simulink library "inverter_model"  (R2024b)
settings: Solver=VariableStepAuto  StartTime=0.0  StopTime=10.0  RelTol=1e-3
settings Model: Creator=jessi  LastModifiedBy=jessi

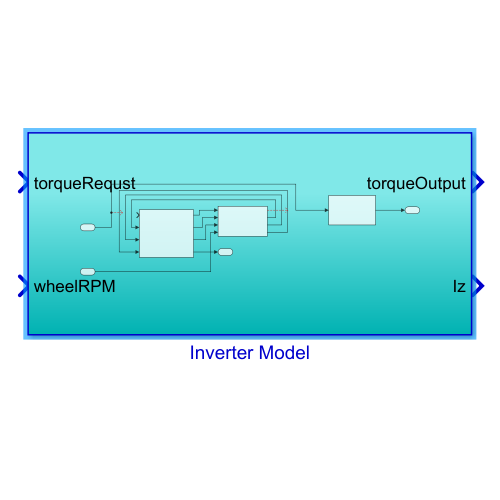
[thumbnail: Simulink's stored preview of the top-level diagram]
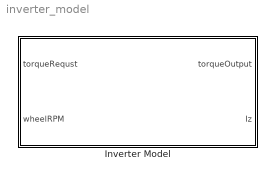
== system inverter_model ==
  Inverter Model : Subsystem

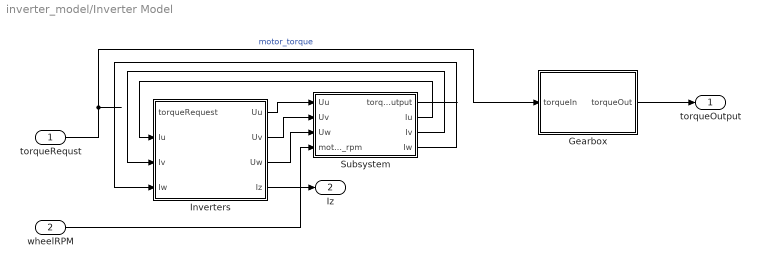
== system inverter_model/Inverter Model ==
  torqueRequst : Inport
  wheelRPM : Inport  Port=2
  Gearbox : Subsystem
  Inverters : Subsystem
  Subsystem : Subsystem
  torqueOutput : Outport
  Iz : Outport  Port=2
  wires:
  torqueRequst/1 -> Gearbox/1(torqueIn)  "motor_torque"
  Subsystem/1(torqueOutput) -> ?
  Inverters/1(Uu) -> Subsystem/1(Uu)
  Inverters/2(Uv) -> Subsystem/2(Uv)
  Inverters/3(Uw) -> Subsystem/3(Uw)
  Subsystem/2(Iu) -> Inverters/2(Iu)
  Subsystem/3(Iv) -> Inverters/3(Iv)
  Subsystem/4(Iw) -> Inverters/4(Iw)
  Inverters/4(Iz) -> Iz/1
  Gearbox/1(torqueOut) -> torqueOutput/1
  wheelRPM/1 -> Subsystem/4(motor_rpm)

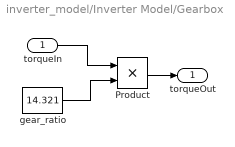
== system inverter_model/Inverter Model/Gearbox ==
  torqueIn : Inport
  Product : Product
  gear_ratio : Constant  Value=14.321
  torqueOut : Outport
  wires:
  torqueIn/1 -> Product/1
  Product/1 -> torqueOut/1
  gear_ratio/1 -> Product/2

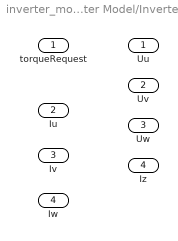
== system inverter_model/Inverter Model/Inverters ==
  torqueRequest : Inport
  Iu : Inport  Port=2
  Iv : Inport  Port=3
  Iw : Inport  Port=4
  Uu : Outport
  Uv : Outport  Port=2
  Uw : Outport  Port=3
  Iz : Outport  Port=4

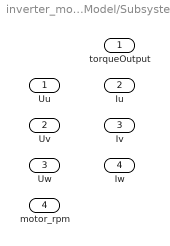
== system inverter_model/Inverter Model/Subsystem ==
  Uu : Inport
  Uv : Inport  Port=2
  Uw : Inport  Port=3
  motor_rpm : Inport  Port=4
  torqueOutput : Outport
  Iu : Outport  Port=2
  Iv : Outport  Port=3
  Iw : Outport  Port=4
